simulink model "One_D_ball_Plate"  (R2020a)
settings: Solver=VariableStepAuto  StartTime=0.0  StopTime=10.0  RelTol=1e-3
model workspace (MAT data in the model file):
  J = Simulink.Parameter
  J.Value = 9.9e-06
  J.DataType = 'auto'
  J.DocUnits = 'kg*m^2'
  J.Dimensions = [1 1]
  L = Simulink.Parameter
  L.Value = 1
  L.DataType = 'auto'
  L.DocUnits = 'm'
  L.Dimensions = [1 1]
  R = Simulink.Parameter
  R.Value = 0.015
  R.DataType = 'auto'
  R.DocUnits = 'm'
  R.Dimensions = [1 1]
  d = Simulink.Parameter
  d.Value = 0.03
  d.DataType = 'auto'
  d.DocUnits = 'm'
  d.Dimensions = [1 1]
  g = Simulink.Parameter
  g.Value = 9.8
  g.DataType = 'auto'
  g.DocUnits = 'm/s^2'
  g.Dimensions = [1 1]
  m = Simulink.Parameter
  m.Value = 0.11
  m.DataType = 'auto'
  m.DocUnits = 'kg'
  m.Dimensions = [1 1]
values from neighbouring files (symbols this model uses):
  d = 0.03    [Root_Locus.m]
  g = -9.8    [Root_Locus.m]
  J = 9.99e-6    (= 9.99e-06)    [Root_Locus.m]
  L = 1.0    (= 1)    [Root_Locus.m]
  m = 0.111    [Root_Locus.m]
  R = 0.015    [Root_Locus.m]
settings Model: Creator=jgrou  LastModifiedBy=jgrou

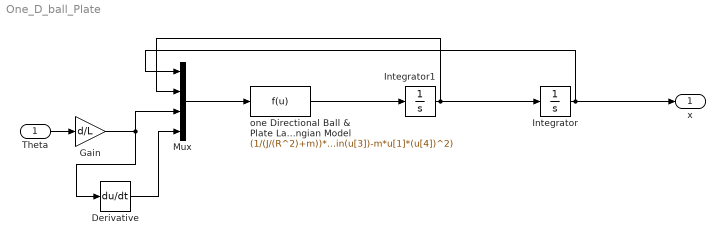
== system One_D_ball_Plate ==
  Theta : Inport
  Derivative : Derivative
  Gain : Gain  Gain=d/L
  Integrator : Integrator
  Integrator1 : Integrator
  Mux : Mux
  one Directional Ball & Plate Lagrangian Model : Fcn  Expr=(1/(J/(R^2)+m))*(m*g*sin(u[3])-m*u[1]*(u[4])^2)
  x : Outport
  wires:
  Theta/1 -> Gain/1
  Gain/1 -> Mux/3, Derivative/1
  one Directional Ball & Plate Lagrangian Model/1 -> Integrator1/1
  Derivative/1 -> Mux/4
  Mux/1 -> one Directional Ball & Plate Lagrangian Model/1
  Integrator/1 -> Mux/1, x/1
  Integrator1/1 -> Mux/2, Integrator/1
